simulink model "Feeder_1"  (Simulink 8.8)
settings: Solver=ode4  StartTime=0.0  StopTime=inf  FixedStep=Ts  RelTol=1e-3  EnableMultiTasking=on
PreLoadFcn:
  | Ts=125e-6;Core_Num = 0; np=1; nq=1; Vmin=.9;
PostLoadFcn:
  | Ts=125e-6;Core_Num = 0; np=1; nq=1; Vmin=.9;
InitFcn:
  | Ts=125e-6;Core_Num = 0; np=1; nq=1; Vmin=.9;
undefined symbols (not defined in the file or in its folder): another_event_name, DiscIntNeverNeededParam, I, j, Left, my_event_name, Right, type, V, X
libraries: powerlib x316, powerlib_meascontrol x227, simulink_extras x78, simulink x25, rtio_generic_c37_118 x22, ssn_lib x9, rtlab x6, powerlib_extras x3, artemis x1, rtio_opalrt_ml605ex1 x1, rtio_spectracom x1, rtio_generic_ethernet x1
(part 3 of 14)

== system Feeder_1/SS_DBUS ==
  DATATX : Inport
  Display : Display
  Ethernet  communication  interface : rtio_generic_ethernet/Ethernet communication interface  ctrl_id=1  nbr_to_remote_endpoint=64  type_to_remote_endpoint=FLOAT  offset_to_remote_endpoint=0  swap_tx=on  nbr_from_remote_endpoint=62  type_from_remote_endpoint=FLOAT  offset_from_remote_endpoint=0  swap_rx=on  exe_name='AsyncEthernet'  nic_name='eth0'  protocol=TCP  tcp_mode=Client  port=6340  remote_ip='10.1.2.2'
  OpComm : rtlab/OpComm  nbport=1  groupe_acq=1  subsys_rate=0  st=0  Synchronization=on  Interpolation=on  Threshold=1.0  Missed_Data=off  Sim_Time=off  Samples=off  dynSigOut=off  from_console=0  warning_done=off  writeOpCommFile=off  Offset=off
  Pulse input : DiscretePulseGenerator  Period=round(1/Ts)  SampleTime=Ts
  Terminator2 : Terminator
  DATARX : Outport
  PQIN : Outport  Port=2
  wires:
  Ethernet  communication  interface/2 -> Terminator2/1
  Pulse input/1 -> Ethernet  communication  interface/1
  DATATX/1 -> OpComm/1
  Ethernet  communication  interface/1 -> PQIN/1, DATARX/1
  OpComm/1 -> Display/1, Ethernet  communication  interface/2

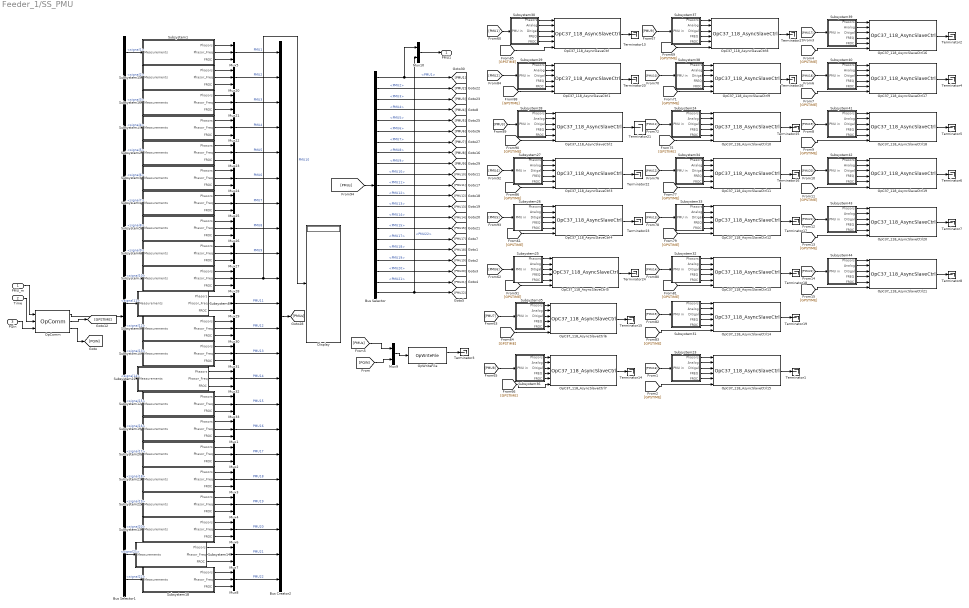
== system Feeder_1/SS_PMU ==
  PMU_m : Inport
  Time : Inport  Port=2
  PQin : Inport  Port=3
  Bus Creator2 : BusCreator  Inputs=22
  Bus Selector : BusSelector  OutputSignals=PMU1,PMU2,PMU3,PMU4,PMU5,PMU6,PMU7,PMU8,PMU9,PMU10,PMU11,PMU12,PMU13,PMU14,PMU15,PMU17,PMU18,PMU19,PMU20,PMU21,PMU22
  Bus Selector1 : BusSelector  OutputSignals=signal1,signal2,signal3,signal4,signal5,signal6,signal7,signal8,signal9,signal10,signal11,signal12,signal13,signal14,signal15,signal16,signal17,signal18,signal19,signal20,signal21,signal22
  Display : Display
  Mux{1..8,20..33} (22 alike) : Mux  Inputs=3
  Mux10 : Mux  Inputs=2
  Mux9 : Mux  Inputs=2
  OpC37_118_AsyncSlaveCtrl : rtio_generic_c37_118/OpC37_118_AsyncSlaveCtrl  dev_id=1  pmu_name='PMU1'  core_nbr=0  exe_name='AsyncC37_118_Slave'  nic_name='eth2'  proto=TCP  udp_port=7501  ip_addr_local='10.1.6.88'  port_local=7518  nominal_freq=60 Hz  data_rate_50=50  data_rate_60=30  timebase=1000000  ts_in=on  cfg_name='pmu_in_cfg.xml'
  OpC37_118_AsyncSlaveCtrl1 : rtio_generic_c37_118/OpC37_118_AsyncSlaveCtrl  dev_id=2  pmu_name='PMU2'  core_nbr=0  exe_name='AsyncC37_118_Slave'  nic_name='eth2'  proto=TCP  udp_port=7502  ip_addr_local='10.1.6.89'  port_local=7519  nominal_freq=60 Hz  data_rate_50=50  data_rate_60=30  timebase=1000000  ts_in=on  cfg_name='pmu_in_cfg.xml'
  OpC37_118_AsyncSlaveCtrl10 : rtio_generic_c37_118/OpC37_118_AsyncSlaveCtrl  dev_id=11  pmu_name='PMU11'  core_nbr=0  exe_name='AsyncC37_118_Slave'  nic_name='eth2'  proto=TCP  udp_port=7511  ip_addr_local='10.1.6.98'  port_local=7528  nominal_freq=60 Hz  data_rate_50=50  data_rate_60=30  timebase=1000000  ts_in=on  cfg_name='pmu_in_cfg.xml'
  OpC37_118_AsyncSlaveCtrl11 : rtio_generic_c37_118/OpC37_118_AsyncSlaveCtrl  dev_id=12  pmu_name='PMU12'  core_nbr=0  exe_name='AsyncC37_118_Slave'  nic_name='eth2'  proto=TCP  udp_port=7512  ip_addr_local='10.1.6.99'  port_local=7529  nominal_freq=60 Hz  data_rate_50=50  data_rate_60=30  timebase=1000000  ts_in=on  cfg_name='pmu_in_cfg.xml'
  OpC37_118_AsyncSlaveCtrl12 : rtio_generic_c37_118/OpC37_118_AsyncSlaveCtrl  dev_id=13  pmu_name='PMU13'  core_nbr=0  exe_name='AsyncC37_118_Slave'  nic_name='eth2'  proto=TCP  udp_port=7513  ip_addr_local='10.1.6.100'  port_local=7530  nominal_freq=60 Hz  data_rate_50=50  data_rate_60=30  timebase=1000000  ts_in=on  cfg_name='pmu_in_cfg.xml'
  OpC37_118_AsyncSlaveCtrl13 : rtio_generic_c37_118/OpC37_118_AsyncSlaveCtrl  dev_id=14  pmu_name='PMU14'  core_nbr=0  exe_name='AsyncC37_118_Slave'  nic_name='eth2'  proto=TCP  udp_port=7514  ip_addr_local='10.1.6.101'  port_local=7531  nominal_freq=60 Hz  data_rate_50=50  data_rate_60=30  timebase=1000000  ts_in=on  cfg_name='pmu_in_cfg.xml'
  OpC37_118_AsyncSlaveCtrl14 : rtio_generic_c37_118/OpC37_118_AsyncSlaveCtrl  dev_id=15  pmu_name='PMU15'  core_nbr=0  exe_name='AsyncC37_118_Slave'  nic_name='eth2'  proto=TCP  udp_port=7515  ip_addr_local='10.1.6.102'  port_local=7532  nominal_freq=60 Hz  data_rate_50=50  data_rate_60=30  timebase=1000000  ts_in=on  cfg_name='pmu_in_cfg.xml'
  OpC37_118_AsyncSlaveCtrl15 : rtio_generic_c37_118/OpC37_118_AsyncSlaveCtrl  dev_id=16  pmu_name='PMU16'  core_nbr=0  exe_name='AsyncC37_118_Slave'  nic_name='eth2'  proto=TCP  udp_port=7515  ip_addr_local='10.1.6.103'  port_local=7533  nominal_freq=60 Hz  data_rate_50=50  data_rate_60=30  timebase=1000000  ts_in=on  cfg_name='pmu_in_cfg.xml'
  OpC37_118_AsyncSlaveCtrl16 : rtio_generic_c37_118/OpC37_118_AsyncSlaveCtrl  dev_id=17  pmu_name='PMU17'  core_nbr=0  exe_name='AsyncC37_118_Slave'  nic_name='eth2'  proto=TCP  udp_port=7515  ip_addr_local='10.1.6.104'  port_local=7534  nominal_freq=60 Hz  data_rate_50=50  data_rate_60=30  timebase=1000000  ts_in=on  cfg_name='pmu_in_cfg.xml'
  OpC37_118_AsyncSlaveCtrl17 : rtio_generic_c37_118/OpC37_118_AsyncSlaveCtrl  dev_id=18  pmu_name='PMU18'  core_nbr=0  exe_name='AsyncC37_118_Slave'  nic_name='eth2'  proto=TCP  udp_port=7515  ip_addr_local='10.1.6.105'  port_local=7535  nominal_freq=60 Hz  data_rate_50=50  data_rate_60=30  timebase=1000000  ts_in=on  cfg_name='pmu_in_cfg.xml'
  OpC37_118_AsyncSlaveCtrl18 : rtio_generic_c37_118/OpC37_118_AsyncSlaveCtrl  dev_id=19  pmu_name='PMU19'  core_nbr=0  exe_name='AsyncC37_118_Slave'  nic_name='eth2'  proto=TCP  udp_port=7515  ip_addr_local='10.1.6.106'  port_local=7536  nominal_freq=60 Hz  data_rate_50=50  data_rate_60=30  timebase=1000000  ts_in=on  cfg_name='pmu_in_cfg.xml'
  OpC37_118_AsyncSlaveCtrl19 : rtio_generic_c37_118/OpC37_118_AsyncSlaveCtrl  dev_id=20  pmu_name='PMU20'  core_nbr=0  exe_name='AsyncC37_118_Slave'  nic_name='eth2'  proto=TCP  udp_port=7515  ip_addr_local='10.1.6.107'  port_local=7537  nominal_freq=60 Hz  data_rate_50=50  data_rate_60=30  timebase=1000000  ts_in=on  cfg_name='pmu_in_cfg.xml'
  OpC37_118_AsyncSlaveCtrl2 : rtio_generic_c37_118/OpC37_118_AsyncSlaveCtrl  dev_id=3  pmu_name='PMU3'  core_nbr=0  exe_name='AsyncC37_118_Slave'  nic_name='eth2'  proto=TCP  udp_port=7503  ip_addr_local='10.1.6.90'  port_local=7520  nominal_freq=60 Hz  data_rate_50=50  data_rate_60=30  timebase=1000000  ts_in=on  cfg_name='pmu_in_cfg.xml'
  OpC37_118_AsyncSlaveCtrl20 : rtio_generic_c37_118/OpC37_118_AsyncSlaveCtrl  dev_id=21  pmu_name='PMU21'  core_nbr=0  exe_name='AsyncC37_118_Slave'  nic_name='eth2'  proto=TCP  udp_port=7515  ip_addr_local='10.1.6.108'  port_local=7538  nominal_freq=60 Hz  data_rate_50=50  data_rate_60=30  timebase=1000000  ts_in=on  cfg_name='pmu_in_cfg.xml'
  OpC37_118_AsyncSlaveCtrl21 : rtio_generic_c37_118/OpC37_118_AsyncSlaveCtrl  dev_id=22  pmu_name='PMU22'  core_nbr=0  exe_name='AsyncC37_118_Slave'  nic_name='eth2'  proto=TCP  udp_port=7515  ip_addr_local='10.1.6.109'  port_local=7539  nominal_freq=60 Hz  data_rate_50=50  data_rate_60=30  timebase=1000000  ts_in=on  cfg_name='pmu_in_cfg.xml'
  OpC37_118_AsyncSlaveCtrl3 : rtio_generic_c37_118/OpC37_118_AsyncSlaveCtrl  dev_id=4  pmu_name='PMU4'  core_nbr=0  exe_name='AsyncC37_118_Slave'  nic_name='eth2'  proto=TCP  udp_port=7504  ip_addr_local='10.1.6.91'  port_local=7521  nominal_freq=60 Hz  data_rate_50=50  data_rate_60=30  timebase=1000000  ts_in=on  cfg_name='pmu_in_cfg.xml'
  OpC37_118_AsyncSlaveCtrl4 : rtio_generic_c37_118/OpC37_118_AsyncSlaveCtrl  dev_id=5  pmu_name='PMU5'  core_nbr=0  exe_name='AsyncC37_118_Slave'  nic_name='eth2'  proto=TCP  udp_port=7505  ip_addr_local='10.1.6.92'  port_local=7522  nominal_freq=60 Hz  data_rate_50=50  data_rate_60=30  timebase=1000000  ts_in=on  cfg_name='pmu_in_cfg.xml'
  OpC37_118_AsyncSlaveCtrl5 : rtio_generic_c37_118/OpC37_118_AsyncSlaveCtrl  dev_id=6  pmu_name='PMU6'  core_nbr=0  exe_name='AsyncC37_118_Slave'  nic_name='eth2'  proto=TCP  udp_port=7506  ip_addr_local='10.1.6.93'  port_local=7523  nominal_freq=60 Hz  data_rate_50=50  data_rate_60=30  timebase=1000000  ts_in=on  cfg_name='pmu_in_cfg.xml'
  OpC37_118_AsyncSlaveCtrl6 : rtio_generic_c37_118/OpC37_118_AsyncSlaveCtrl  dev_id=7  pmu_name='PMU7'  core_nbr=0  exe_name='AsyncC37_118_Slave'  nic_name='eth2'  proto=TCP  udp_port=7507  ip_addr_local='10.1.6.94'  port_local=7524  nominal_freq=60 Hz  data_rate_50=50  data_rate_60=30  timebase=1000000  ts_in=on  cfg_name='pmu_in_cfg.xml'
  OpC37_118_AsyncSlaveCtrl7 : rtio_generic_c37_118/OpC37_118_AsyncSlaveCtrl  dev_id=8  pmu_name='PMU8'  core_nbr=0  exe_name='AsyncC37_118_Slave'  nic_name='eth2'  proto=TCP  udp_port=7508  ip_addr_local='10.1.6.95'  port_local=7525  nominal_freq=60 Hz  data_rate_50=50  data_rate_60=30  timebase=1000000  ts_in=on  cfg_name='pmu_in_cfg.xml'
  OpC37_118_AsyncSlaveCtrl8 : rtio_generic_c37_118/OpC37_118_AsyncSlaveCtrl  dev_id=9  pmu_name='PMU9'  core_nbr=0  exe_name='AsyncC37_118_Slave'  nic_name='eth2'  proto=TCP  udp_port=7509  ip_addr_local='10.1.6.96'  port_local=7526  nominal_freq=60 Hz  data_rate_50=50  data_rate_60=30  timebase=1000000  ts_in=on  cfg_name='pmu_in_cfg.xml'
  OpC37_118_AsyncSlaveCtrl9 : rtio_generic_c37_118/OpC37_118_AsyncSlaveCtrl  dev_id=10  pmu_name='PMU10'  core_nbr=0  exe_name='AsyncC37_118_Slave'  nic_name='eth2'  proto=TCP  udp_port=7510  ip_addr_local='10.1.6.97'  port_local=7527  nominal_freq=60 Hz  data_rate_50=50  data_rate_60=30  timebase=1000000  ts_in=on  cfg_name='pmu_in_cfg.xml'
  OpComm : rtlab/OpComm  nbport=3  groupe_acq=1  subsys_rate=0  st=0  Synchronization=on  Interpolation=on  Threshold=1.0  Missed_Data=off  Sim_Time=off  Samples=off  dynSigOut=off  from_console=0  warning_done=off  writeOpCommFile=off  Offset=off
  OpWriteFile : rtlab/DataLogging/OpWriteFile  Static_File=on  varname=Baseline  Filename=Energise.mat  rtpath='./'  nrtpath='E:\Models\LOHO13_GT_DBUS\Results\Testdata'  Acq_Group=30  file_size=38092800  write_offline=off  Sim_Mode=off  Nb_Samples=800  Buffer_size=2374400
      settings: Decimation=10000
  Subsystem1 : Subsystem
  Subsystem10 : Subsystem
  Subsystem11 : Subsystem
  Subsystem12 : Subsystem
  Subsystem13 : Subsystem
  Subsystem14 : Subsystem
  Subsystem15 : Subsystem
  Subsystem16 : Subsystem
  Subsystem17 : Subsystem
  Subsystem18 : Subsystem
  Subsystem19 : Subsystem
  Subsystem2 : Subsystem
  Subsystem20 : Subsystem
  Subsystem21 : Subsystem
  Subsystem22 : Subsystem
  Subsystem23 : Subsystem
  Subsystem24 : Subsystem
  Subsystem25 : Subsystem
  Subsystem26 : Subsystem
  Subsystem27 : Subsystem
  Subsystem28 : Subsystem
  Subsystem29 : Subsystem
  Subsystem3 : Subsystem
  Subsystem30 : Subsystem
  Subsystem31 : Subsystem
  Subsystem32 : Subsystem
  Subsystem33 : Subsystem
  Subsystem34 : Subsystem
  Subsystem35 : Subsystem
  Subsystem36 : Subsystem
  Subsystem37 : Subsystem
  Subsystem38 : Subsystem
  Subsystem39 : Subsystem
  Subsystem4 : Subsystem
  Subsystem40 : Subsystem
  Subsystem41 : Subsystem
  Subsystem42 : Subsystem
  Subsystem43 : Subsystem
  Subsystem44 : Subsystem
  Subsystem5 : Subsystem
  Subsystem6 : Subsystem
  Subsystem7 : Subsystem
  Subsystem8 : Subsystem
  Subsystem9 : Subsystem
  Terminator{1..8,13..27} (23 alike) : Terminator
  PMU1 : Outport
  wires:
  [GPSTIME] -> OpC37_118_AsyncSlaveCtrl/6
  [GPSTIME] -> OpC37_118_AsyncSlaveCtrl1/6
  [GPSTIME] -> OpC37_118_AsyncSlaveCtrl2/6
  [GPSTIME] -> OpC37_118_AsyncSlaveCtrl3/6
  [GPSTIME] -> OpC37_118_AsyncSlaveCtrl4/6
  [GPSTIME] -> OpC37_118_AsyncSlaveCtrl5/6
  [GPSTIME] -> OpC37_118_AsyncSlaveCtrl6/6
  [GPSTIME] -> OpC37_118_AsyncSlaveCtrl7/6
  [GPSTIME] -> OpC37_118_AsyncSlaveCtrl8/6
  [GPSTIME] -> OpC37_118_AsyncSlaveCtrl9/6
  [GPSTIME] -> OpC37_118_AsyncSlaveCtrl10/6
  [GPSTIME] -> OpC37_118_AsyncSlaveCtrl11/6
  [GPSTIME] -> OpC37_118_AsyncSlaveCtrl12/6
  [GPSTIME] -> OpC37_118_AsyncSlaveCtrl13/6
  [GPSTIME] -> OpC37_118_AsyncSlaveCtrl14/6
  Subsystem31/1(Phasors) -> OpC37_118_AsyncSlaveCtrl14/1
  Subsystem31/2(Analog) -> OpC37_118_AsyncSlaveCtrl14/2
  Subsystem31/3(Ditigal) -> OpC37_118_AsyncSlaveCtrl14/3
  Subsystem31/4(FREQ) -> OpC37_118_AsyncSlaveCtrl14/4
  Subsystem31/5(FROC) -> OpC37_118_AsyncSlaveCtrl14/5
  [PMU15] -> Subsystem31/1(PMU in)
  Subsystem32/1(Phasors) -> OpC37_118_AsyncSlaveCtrl13/1
  Subsystem32/2(Analog) -> OpC37_118_AsyncSlaveCtrl13/2
  Subsystem32/3(Ditigal) -> OpC37_118_AsyncSlaveCtrl13/3
  Subsystem32/4(FREQ) -> OpC37_118_AsyncSlaveCtrl13/4
  Subsystem32/5(FROC) -> OpC37_118_AsyncSlaveCtrl13/5
  [PMU14] -> Subsystem32/1(PMU in)
  Subsystem33/1(Phasors) -> OpC37_118_AsyncSlaveCtrl12/1
  Subsystem33/2(Analog) -> OpC37_118_AsyncSlaveCtrl12/2
  Subsystem33/3(Ditigal) -> OpC37_118_AsyncSlaveCtrl12/3
  Subsystem33/4(FREQ) -> OpC37_118_AsyncSlaveCtrl12/4
  Subsystem33/5(FROC) -> OpC37_118_AsyncSlaveCtrl12/5
  [PMU13] -> Subsystem33/1(PMU in)
  Subsystem34/1(Phasors) -> OpC37_118_AsyncSlaveCtrl11/1
  Subsystem34/2(Analog) -> OpC37_118_AsyncSlaveCtrl11/2
  Subsystem34/3(Ditigal) -> OpC37_118_AsyncSlaveCtrl11/3
  Subsystem34/4(FREQ) -> OpC37_118_AsyncSlaveCtrl11/4
  Subsystem34/5(FROC) -> OpC37_118_AsyncSlaveCtrl11/5
  [PMU12] -> Subsystem34/1(PMU in)
  Subsystem35/1(Phasors) -> OpC37_118_AsyncSlaveCtrl6/1
  Subsystem35/2(Analog) -> OpC37_118_AsyncSlaveCtrl6/2
  Subsystem35/3(Ditigal) -> OpC37_118_AsyncSlaveCtrl6/3
  Subsystem35/4(FREQ) -> OpC37_118_AsyncSlaveCtrl6/4
  Subsystem35/5(FROC) -> OpC37_118_AsyncSlaveCtrl6/5
  [PMU7] -> Subsystem35/1(PMU in)
  Subsystem36/1(Phasors) -> OpC37_118_AsyncSlaveCtrl7/1
  Subsystem36/2(Analog) -> OpC37_118_AsyncSlaveCtrl7/2
  Subsystem36/3(Ditigal) -> OpC37_118_AsyncSlaveCtrl7/3
  Subsystem36/4(FREQ) -> OpC37_118_AsyncSlaveCtrl7/4
  Subsystem36/5(FROC) -> OpC37_118_AsyncSlaveCtrl7/5
  [PMU8] -> Subsystem36/1(PMU in)
  Subsystem37/1(Phasors) -> OpC37_118_AsyncSlaveCtrl8/1
  Subsystem37/2(Analog) -> OpC37_118_AsyncSlaveCtrl8/2
  Subsystem37/3(Ditigal) -> OpC37_118_AsyncSlaveCtrl8/3
  Subsystem37/4(FREQ) -> OpC37_118_AsyncSlaveCtrl8/4
  Subsystem37/5(FROC) -> OpC37_118_AsyncSlaveCtrl8/5
  [PMU9] -> Subsystem37/1(PMU in)
  Subsystem38/1(Phasors) -> OpC37_118_AsyncSlaveCtrl9/1
  Subsystem38/2(Analog) -> OpC37_118_AsyncSlaveCtrl9/2
  Subsystem38/3(Ditigal) -> OpC37_118_AsyncSlaveCtrl9/3
  Subsystem38/4(FREQ) -> OpC37_118_AsyncSlaveCtrl9/4
  Subsystem38/5(FROC) -> OpC37_118_AsyncSlaveCtrl9/5
  [PMU10] -> Subsystem38/1(PMU in)
  Subsystem24/1(Phasors) -> OpC37_118_AsyncSlaveCtrl10/1
  Subsystem24/2(Analog) -> OpC37_118_AsyncSlaveCtrl10/2
  Subsystem24/3(Ditigal) -> OpC37_118_AsyncSlaveCtrl10/3
  Subsystem24/4(FREQ) -> OpC37_118_AsyncSlaveCtrl10/4
  Subsystem24/5(FROC) -> OpC37_118_AsyncSlaveCtrl10/5
  [PMU11] -> Subsystem24/1(PMU in)
  Subsystem25/1(Phasors) -> OpC37_118_AsyncSlaveCtrl5/1
  Subsystem25/2(Analog) -> OpC37_118_AsyncSlaveCtrl5/2
  Subsystem25/3(Ditigal) -> OpC37_118_AsyncSlaveCtrl5/3
  Subsystem25/4(FREQ) -> OpC37_118_AsyncSlaveCtrl5/4
  Subsystem25/5(FROC) -> OpC37_118_AsyncSlaveCtrl5/5
  [PMU6] -> Subsystem25/1(PMU in)
  Subsystem26/1(Phasors) -> OpC37_118_AsyncSlaveCtrl4/1
  Subsystem26/2(Analog) -> OpC37_118_AsyncSlaveCtrl4/2
  Subsystem26/3(Ditigal) -> OpC37_118_AsyncSlaveCtrl4/3
  Subsystem26/4(FREQ) -> OpC37_118_AsyncSlaveCtrl4/4
  Subsystem26/5(FROC) -> OpC37_118_AsyncSlaveCtrl4/5
  [PMU5] -> Subsystem26/1(PMU in)
  Subsystem27/1(Phasors) -> OpC37_118_AsyncSlaveCtrl3/1
  Subsystem27/2(Analog) -> OpC37_118_AsyncSlaveCtrl3/2
  Subsystem27/3(Ditigal) -> OpC37_118_AsyncSlaveCtrl3/3
  Subsystem27/4(FREQ) -> OpC37_118_AsyncSlaveCtrl3/4
  Subsystem27/5(FROC) -> OpC37_118_AsyncSlaveCtrl3/5
  [PMU4] -> Subsystem27/1(PMU in)
  Subsystem28/1(Phasors) -> OpC37_118_AsyncSlaveCtrl2/1
  Subsystem28/2(Analog) -> OpC37_118_AsyncSlaveCtrl2/2
  Subsystem28/3(Ditigal) -> OpC37_118_AsyncSlaveCtrl2/3
  Subsystem28/4(FREQ) -> OpC37_118_AsyncSlaveCtrl2/4
  Subsystem28/5(FROC) -> OpC37_118_AsyncSlaveCtrl2/5
  [PMU3] -> Subsystem28/1(PMU in)
  Subsystem29/1(Phasors) -> OpC37_118_AsyncSlaveCtrl1/1
  Subsystem29/2(Analog) -> OpC37_118_AsyncSlaveCtrl1/2
  Subsystem29/3(Ditigal) -> OpC37_118_AsyncSlaveCtrl1/3
  Subsystem29/4(FREQ) -> OpC37_118_AsyncSlaveCtrl1/4
  Subsystem29/5(FROC) -> OpC37_118_AsyncSlaveCtrl1/5
  [PMU2] -> Subsystem29/1(PMU in)
  Subsystem30/1(Phasors) -> OpC37_118_AsyncSlaveCtrl/1
  Subsystem30/2(Analog) -> OpC37_118_AsyncSlaveCtrl/2
  Subsystem30/3(Ditigal) -> OpC37_118_AsyncSlaveCtrl/3
  Subsystem30/4(FREQ) -> OpC37_118_AsyncSlaveCtrl/4
  Subsystem30/5(FROC) -> OpC37_118_AsyncSlaveCtrl/5
  [PMU1] -> Subsystem30/1(PMU in)
  Bus Selector/2 -> [PMU2]  "<PMU2>"
  Bus Selector/3 -> [PMU3]  "<PMU3>"
  Bus Selector/5 -> [PMU5]  "<PMU5>"
  Bus Selector/7 -> [PMU7]  "<PMU7>"
  Bus Selector/9 -> [PMU9]  "<PMU9>"
  Bus Selector/11 -> [PMU11]  "<PMU11>"
  Bus Selector/13 -> [PMU13]  "<PMU13>"
  Bus Selector/15 -> [PMU15]  "<PMU15>"
  OpC37_118_AsyncSlaveCtrl/1 -> Terminator13/1
  OpC37_118_AsyncSlaveCtrl1/1 -> Terminator20/1
  OpC37_118_AsyncSlaveCtrl2/1 -> Terminator21/1
  OpC37_118_AsyncSlaveCtrl3/1 -> Terminator22/1
  OpC37_118_AsyncSlaveCtrl4/1 -> Terminator23/1
  OpC37_118_AsyncSlaveCtrl5/1 -> Terminator24/1
  OpC37_118_AsyncSlaveCtrl10/1 -> Terminator25/1
  OpC37_118_AsyncSlaveCtrl9/1 -> Terminator26/1
  OpC37_118_AsyncSlaveCtrl8/1 -> Terminator27/1
  OpC37_118_AsyncSlaveCtrl7/1 -> Terminator14/1
  OpC37_118_AsyncSlaveCtrl6/1 -> Terminator15/1
  OpC37_118_AsyncSlaveCtrl11/1 -> Terminator16/1
  OpC37_118_AsyncSlaveCtrl12/1 -> Terminator17/1
  OpC37_118_AsyncSlaveCtrl13/1 -> Terminator18/1
  OpC37_118_AsyncSlaveCtrl14/1 -> Terminator19/1
  PMU_m/1 -> OpComm/1
  Time/1 -> OpComm/2
  OpComm/2 -> [GPSTIME]
  Subsystem1/1(Phasors) -> Mux5/1
  Subsystem1/2(Phasor_Freq) -> Mux5/2
  Subsystem1/3(FROC) -> Mux5/3
  Subsystem15/1(Phasors) -> Mux20/1
  Subsystem15/2(Phasor_Freq) -> Mux20/2
  Subsystem15/3(FROC) -> Mux20/3
  Subsystem16/1(Phasors) -> Mux21/1
  Mux33/1 -> Bus Creator2/15  "PMU15"
  Mux32/1 -> Bus Creator2/14  "PMU14"
  Mux31/1 -> Bus Creator2/13  "PMU13"
  Mux30/1 -> Bus Creator2/12  "PMU12"
  Mux29/1 -> Bus Creator2/11  "PMU11"
  Mux5/1 -> Bus Creator2/1  "PMU1"
  Mux20/1 -> Bus Creator2/2  "PMU2"
  Mux21/1 -> Bus Creator2/3  "PMU3"
  Mux22/1 -> Bus Creator2/4  "PMU4"
  Mux23/1 -> Bus Creator2/5  "PMU5"
  Mux24/1 -> Bus Creator2/6  "PMU6"
  Mux25/1 -> Bus Creator2/7  "PMU7"
  Mux27/1 -> Bus Creator2/9  "PMU9"
  Mux28/1 -> Display/1, Bus Creator2/10  "PMU10"
  Mux26/1 -> Bus Creator2/8  "PMU8"
  Subsystem16/2(Phasor_Freq) -> Mux21/2
  Subsystem16/3(FROC) -> Mux21/3
  Subsystem17/1(Phasors) -> Mux22/1
  Subsystem17/2(Phasor_Freq) -> Mux22/2
  Subsystem17/3(FROC) -> Mux22/3
  Subsystem2/1(Phasors) -> Mux23/1
  Subsystem2/3(FROC) -> Mux23/3
  Subsystem2/2(Phasor_Freq) -> Mux23/2
  Subsystem3/1(Phasors) -> Mux24/1
  Subsystem3/2(Phasor_Freq) -> Mux24/2
  Subsystem3/3(FROC) -> Mux24/3
  Subsystem4/1(Phasors) -> Mux25/1
  Subsystem4/2(Phasor_Freq) -> Mux25/2
  Subsystem4/3(FROC) -> Mux25/3
  Subsystem5/1(Phasors) -> Mux26/1
  Subsystem5/2(Phasor_Freq) -> Mux26/2
  Subsystem5/3(FROC) -> Mux26/3
  Subsystem6/1(Phasors) -> Mux27/1
  Subsystem6/2(Phasor_Freq) -> Mux27/2
  Subsystem6/3(FROC) -> Mux27/3
  Subsystem7/1(Phasors) -> Mux28/1
  Subsystem7/2(Phasor_Freq) -> Mux28/2
  Subsystem7/3(FROC) -> Mux28/3
  Subsystem8/1(Phasors) -> Mux29/1
  Subsystem8/2(Phasor_Freq) -> Mux29/2
  Subsystem8/3(FROC) -> Mux29/3
  Subsystem9/1(Phasors) -> Mux30/1
  Subsystem9/2(Phasor_Freq) -> Mux30/2
  Subsystem9/3(FROC) -> Mux30/3
  Subsystem10/1(Phasors) -> Mux31/1
  Subsystem10/2(Phasor_Freq) -> Mux31/2
  Subsystem10/3(FROC) -> Mux31/3
  Subsystem11/1(Phasors) -> Mux32/1
  Subsystem11/2(Phasor_Freq) -> Mux32/2
  Subsystem11/3(FROC) -> Mux32/3
  Subsystem12/1(Phasors) -> Mux33/1
  Subsystem12/2(Phasor_Freq) -> Mux33/2
  Subsystem12/3(FROC) -> Mux33/3
  Bus Selector1/1 -> Subsystem1/1(Measurements)  "<signal1>"
  Bus Selector1/2 -> Subsystem15/1(Measurements)  "<signal2>"
  Bus Selector1/3 -> Subsystem16/1(Measurements)  "<signal3>"
  Bus Selector1/4 -> Subsystem17/1(Measurements)  "<signal4>"
  Bus Selector1/5 -> Subsystem2/1(Measurements)  "<signal5>"
  Bus Selector1/6 -> Subsystem3/1(Measurements)  "<signal6>"
  Bus Selector1/7 -> Subsystem4/1(Measurements)  "<signal7>"
  Bus Selector1/8 -> Subsystem5/1(Measurements)  "<signal8>"
  Bus Selector1/9 -> Subsystem6/1(Measurements)  "<signal9>"
  Bus Selector1/10 -> Subsystem7/1(Measurements)  "<signal10>"
  Bus Selector1/11 -> Subsystem8/1(Measurements)  "<signal11>"
  Bus Selector1/12 -> Subsystem9/1(Measurements)  "<signal12>"
  Bus Selector1/13 -> Subsystem10/1(Measurements)  "<signal13>"
  Bus Selector1/14 -> Subsystem11/1(Measurements)  "<signal14>"
  Bus Selector1/15 -> Subsystem12/1(Measurements)  "<signal15>"
  OpComm/1 -> Bus Selector1/1
  Bus Creator2/1 -> [PMUs]
  [PMUs] -> Bus Selector/1
  Bus Selector/4 -> [PMU4]  "<PMU4>"
  Bus Selector/6 -> [PMU6]  "<PMU6>"
  Bus Selector/8 -> [PMU8]  "<PMU8>"
  Bus Selector/10 -> [PMU10]  "<PMU10>"
  Bus Selector/12 -> [PMU12]  "<PMU12>"
  Bus Selector/14 -> [PMU14]  "<PMU14>"
  Bus Selector/1 -> Mux10/1, [PMU1]  "<PMU1>"
  OpWriteFile/1 -> Terminator3/1
  Bus Selector1/22 -> Subsystem18/1(Measurements)  "<signal22>"
  Bus Selector1/21 -> Subsystem14/1(Measurements)  "<signal21>"
  Bus Selector1/20 -> Subsystem13/1(Measurements)  "<signal20>"
  Bus Selector1/19 -> Subsystem22/1(Measurements)  "<signal19>"
  Bus Selector1/18 -> Subsystem21/1(Measurements)  "<signal18>"
  Bus Selector1/17 -> Subsystem20/1(Measurements)  "<signal17>"
  Bus Selector1/16 -> Subsystem19/1(Measurements)  "<signal16>"
  Mux8/1 -> Bus Creator2/22  "PMU22"
  Mux7/1 -> Bus Creator2/21  "PMU21"
  Mux6/1 -> Bus Creator2/20  "PMU20"
  Mux4/1 -> Bus Creator2/19  "PMU19"
  Mux3/1 -> Bus Creator2/18  "PMU18"
  Mux1/1 -> Bus Creator2/16  "PMU16"
  Mux2/1 -> Bus Creator2/17  "PMU17"
  Subsystem19/1(Phasors) -> Mux1/1
  Subsystem19/2(Phasor_Freq) -> Mux1/2
  Subsystem19/3(FROC) -> Mux1/3
  Subsystem20/1(Phasors) -> Mux2/1
  Subsystem20/2(Phasor_Freq) -> Mux2/2
  Subsystem20/3(FROC) -> Mux2/3
  Subsystem21/1(Phasors) -> Mux3/1
  Subsystem21/2(Phasor_Freq) -> Mux3/2
  Subsystem21/3(FROC) -> Mux3/3
  Subsystem22/1(Phasors) -> Mux4/1
  Subsystem22/2(Phasor_Freq) -> Mux4/2
  Subsystem22/3(FROC) -> Mux4/3
  Subsystem13/1(Phasors) -> Mux6/1
  Subsystem13/2(Phasor_Freq) -> Mux6/2
  Subsystem13/3(FROC) -> Mux6/3
  Subsystem14/1(Phasors) -> Mux7/1
  Subsystem14/2(Phasor_Freq) -> Mux7/2
  Subsystem14/3(FROC) -> Mux7/3
  Subsystem18/1(Phasors) -> Mux8/1
  Subsystem18/2(Phasor_Freq) -> Mux8/2
  Subsystem18/3(FROC) -> Mux8/3
  [GPSTIME] -> OpC37_118_AsyncSlaveCtrl15/6
  Subsystem23/1(Phasors) -> OpC37_118_AsyncSlaveCtrl15/1
  Subsystem23/2(Analog) -> OpC37_118_AsyncSlaveCtrl15/2
  Subsystem23/3(Ditigal) -> OpC37_118_AsyncSlaveCtrl15/3
  Subsystem23/4(FREQ) -> OpC37_118_AsyncSlaveCtrl15/4
  Subsystem23/5(FROC) -> OpC37_118_AsyncSlaveCtrl15/5
  [PMU16] -> Subsystem23/1(PMU in)
  OpC37_118_AsyncSlaveCtrl15/1 -> Terminator1/1
  [GPSTIME] -> OpC37_118_AsyncSlaveCtrl16/6
  Subsystem39/1(Phasors) -> OpC37_118_AsyncSlaveCtrl16/1
  Subsystem39/2(Analog) -> OpC37_118_AsyncSlaveCtrl16/2
  Subsystem39/3(Ditigal) -> OpC37_118_AsyncSlaveCtrl16/3
  Subsystem39/4(FREQ) -> OpC37_118_AsyncSlaveCtrl16/4
  Subsystem39/5(FROC) -> OpC37_118_AsyncSlaveCtrl16/5
  [PMU17] -> Subsystem39/1(PMU in)
  OpC37_118_AsyncSlaveCtrl16/1 -> Terminator2/1
  [GPSTIME] -> OpC37_118_AsyncSlaveCtrl17/6
  Subsystem40/1(Phasors) -> OpC37_118_AsyncSlaveCtrl17/1
  Subsystem40/2(Analog) -> OpC37_118_AsyncSlaveCtrl17/2
  Subsystem40/3(Ditigal) -> OpC37_118_AsyncSlaveCtrl17/3
  Subsystem40/4(FREQ) -> OpC37_118_AsyncSlaveCtrl17/4
  Subsystem40/5(FROC) -> OpC37_118_AsyncSlaveCtrl17/5
  [PMU18] -> Subsystem40/1(PMU in)
  OpC37_118_AsyncSlaveCtrl17/1 -> Terminator4/1
  [GPSTIME] -> OpC37_118_AsyncSlaveCtrl18/6
  Subsystem41/2(Analog) -> OpC37_118_AsyncSlaveCtrl18/2
  Subsystem41/3(Ditigal) -> OpC37_118_AsyncSlaveCtrl18/3
  Subsystem41/4(FREQ) -> OpC37_118_AsyncSlaveCtrl18/4
  Subsystem41/5(FROC) -> OpC37_118_AsyncSlaveCtrl18/5
  [PMU19] -> Subsystem41/1(PMU in)
  OpC37_118_AsyncSlaveCtrl18/1 -> Terminator5/1
  [GPSTIME] -> OpC37_118_AsyncSlaveCtrl19/6
  Subsystem42/2(Analog) -> OpC37_118_AsyncSlaveCtrl19/2
  Subsystem42/3(Ditigal) -> OpC37_118_AsyncSlaveCtrl19/3
  Subsystem42/4(FREQ) -> OpC37_118_AsyncSlaveCtrl19/4
  Subsystem42/5(FROC) -> OpC37_118_AsyncSlaveCtrl19/5
  [PMU20] -> Subsystem42/1(PMU in)
  OpC37_118_AsyncSlaveCtrl19/1 -> Terminator6/1
  Subsystem42/1(Phasors) -> OpC37_118_AsyncSlaveCtrl19/1
  Subsystem41/1(Phasors) -> OpC37_118_AsyncSlaveCtrl18/1
  [GPSTIME] -> OpC37_118_AsyncSlaveCtrl20/6
  Subsystem43/2(Analog) -> OpC37_118_AsyncSlaveCtrl20/2
  Subsystem43/3(Ditigal) -> OpC37_118_AsyncSlaveCtrl20/3
  Subsystem43/4(FREQ) -> OpC37_118_AsyncSlaveCtrl20/4
  Subsystem43/5(FROC) -> OpC37_118_AsyncSlaveCtrl20/5
  [PMU21] -> Subsystem43/1(PMU in)
  OpC37_118_AsyncSlaveCtrl20/1 -> Terminator7/1
  Subsystem43/1(Phasors) -> OpC37_118_AsyncSlaveCtrl20/1
  [GPSTIME] -> OpC37_118_AsyncSlaveCtrl21/6
  Subsystem44/2(Analog) -> OpC37_118_AsyncSlaveCtrl21/2
  Subsystem44/3(Ditigal) -> OpC37_118_AsyncSlaveCtrl21/3
  Subsystem44/4(FREQ) -> OpC37_118_AsyncSlaveCtrl21/4
  Subsystem44/5(FROC) -> OpC37_118_AsyncSlaveCtrl21/5
  [PMU22] -> Subsystem44/1(PMU in)
  OpC37_118_AsyncSlaveCtrl21/1 -> Terminator8/1
  Subsystem44/1(Phasors) -> OpC37_118_AsyncSlaveCtrl21/1
  Bus Selector/21 -> Mux10/2, [PMU22]  "<PMU22>"
  Bus Selector/20 -> [PMU21]  "<PMU21>"
  Bus Selector/19 -> [PMU20]  "<PMU20>"
  Bus Selector/18 -> [PMU19]  "<PMU19>"
  Bus Selector/17 -> [PMU18]  "<PMU18>"
  Bus Selector/16 -> [PMU17]  "<PMU17>"
  [PMUs] -> Mux9/1
  Mux9/1 -> OpWriteFile/1
  PQin/1 -> OpComm/3
  OpComm/3 -> [PQIN]
  [PQIN] -> Mux9/2
  Mux10/1 -> PMU1/1

== system Feeder_1/SM_NG/Dynamic Load BCDC2 ==
  P : Inport
  Q : Inport  Port=2
  Ground27 : powerlib/Elements/Ground  LConnTagsString=a
  Single-Phase Dynamic Load1 : Subsystem  DialogController=POWERSYS.PowerSysDialog  mask(Single-Phase Dynamic Load){NominalVoltage=|, ActiveReactivePowers=[934247.1199 467237.5312], PositiveSequence=[1 0], ExternalControl=on, NpNq=[np nq], TimeConstants=[0  0  0  0], MinimumVoltage=Vmin, LoadFlowParameters=[4,0,0,0,0]}
      mask NominalVoltage=|
      | [7967.4337
      | 60]
      mask prompts: NominalVoltage "Nominal voltage and frequency  [Vn(Vrms) fn(Hz)]:"; ActiveReactivePowers "Active and reactive power at initial voltage [Po(W) Qo(var)]:"; PositiveSequence "Initial voltage Vo [Mag(pu) Phase (deg.)]:"; ExternalControl "External control of PQ"; NpNq "Parameters [ np  nq ]:"; TimeConstants "Time constants [Tp1 Tp2 Tq1 Tq2]  (s):"; MinimumVoltage "Minimum voltage Vmin (pu):"; LoadFlowParameters "Load Flow parameters"
      mask help:
      | Implements a single-phase dynamic load. Active  power P and reactive
      | power Q absorbed by the load vary as function of voltage V  according to the
      | following equations:
      |
      |   If V>Vmin, P and Q vary as follows:
      |        P = Po * (V/Vo)^np * (1+Tp1.s)/(1+Tp2.s)
      |        Q = Qo * (V/Vo)^nq * (1+Tq1.s)/(1+Tq2.s)
      |   if V<Vmin
      |      Same equations with np=nq=2 (constant impedance load)
      mask init: same as Feeder_1/SM_NG/Single-Phase Dynamic Load32
      mask Help: helpview(psbhelp)
      mask Callback ExternalControl: powericon('ThreePhaseDynamicLoadCback',gcb);
      mask Display:
      | plot(-45,-45,45,45,[0,9,18,24,29,30,29,24,18,9,0,-9,-18,-24,-29,-30,-29,-24,-18,-9,0]*.9,[30,29,24,18,9,0,-9,-18,-24,-29,-30,-29,-24,-18,-9,0,9,18,24,29,30]*.9)
      | plot([0,0,10,0,-10,0]*1.1,[15,-5,-5,-15,-5,-5]*1.1)
  Single-Phase Dynamic Load2 : Subsystem  DialogController=POWERSYS.PowerSysDialog  mask(Single-Phase Dynamic Load){NominalVoltage=|, ActiveReactivePowers=[586764.5672 402164.5376], PositiveSequence=[1 0], ExternalControl=on, NpNq=[np nq], TimeConstants=[0  0  0  0], MinimumVoltage=Vmin, LoadFlowParameters=[4,0,0,0,0]}
      mask NominalVoltage=|
      | [7967.4337
      | 60]
      mask prompts: NominalVoltage "Nominal voltage and frequency  [Vn(Vrms) fn(Hz)]:"; ActiveReactivePowers "Active and reactive power at initial voltage [Po(W) Qo(var)]:"; PositiveSequence "Initial voltage Vo [Mag(pu) Phase (deg.)]:"; ExternalControl "External control of PQ"; NpNq "Parameters [ np  nq ]:"; TimeConstants "Time constants [Tp1 Tp2 Tq1 Tq2]  (s):"; MinimumVoltage "Minimum voltage Vmin (pu):"; LoadFlowParameters "Load Flow parameters"
      mask help:
      | Implements a single-phase dynamic load. Active  power P and reactive
      | power Q absorbed by the load vary as function of voltage V  according to the
      | following equations:
      |
      |   If V>Vmin, P and Q vary as follows:
      |        P = Po * (V/Vo)^np * (1+Tp1.s)/(1+Tp2.s)
      |        Q = Qo * (V/Vo)^nq * (1+Tq1.s)/(1+Tq2.s)
      |   if V<Vmin
      |      Same equations with np=nq=2 (constant impedance load)
      mask init: same as Feeder_1/SM_NG/Single-Phase Dynamic Load32
      mask Help: helpview(psbhelp)
      mask Callback ExternalControl: powericon('ThreePhaseDynamicLoadCback',gcb);
      mask Display:
      | plot(-45,-45,45,45,[0,9,18,24,29,30,29,24,18,9,0,-9,-18,-24,-29,-30,-29,-24,-18,-9,0]*.9,[30,29,24,18,9,0,-9,-18,-24,-29,-30,-29,-24,-18,-9,0,9,18,24,29,30]*.9)
      | plot([0,0,10,0,-10,0]*1.1,[15,-5,-5,-15,-5,-5]*1.1)
  Single-Phase Dynamic Load9 : Subsystem  DialogController=POWERSYS.PowerSysDialog  mask(Single-Phase Dynamic Load){NominalVoltage=|, ActiveReactivePowers=[473340.7231 336359.2548], PositiveSequence=[1 0], ExternalControl=on, NpNq=[np nq], TimeConstants=[0  0  0  0], MinimumVoltage=Vmin, LoadFlowParameters=[4,0,0,0,0]}
      mask NominalVoltage=|
      | [7967.4337
      | 60]
      mask prompts: NominalVoltage "Nominal voltage and frequency  [Vn(Vrms) fn(Hz)]:"; ActiveReactivePowers "Active and reactive power at initial voltage [Po(W) Qo(var)]:"; PositiveSequence "Initial voltage Vo [Mag(pu) Phase (deg.)]:"; ExternalControl "External control of PQ"; NpNq "Parameters [ np  nq ]:"; TimeConstants "Time constants [Tp1 Tp2 Tq1 Tq2]  (s):"; MinimumVoltage "Minimum voltage Vmin (pu):"; LoadFlowParameters "Load Flow parameters"
      mask help:
      | Implements a single-phase dynamic load. Active  power P and reactive
      | power Q absorbed by the load vary as function of voltage V  according to the
      | following equations:
      |
      |   If V>Vmin, P and Q vary as follows:
      |        P = Po * (V/Vo)^np * (1+Tp1.s)/(1+Tp2.s)
      |        Q = Qo * (V/Vo)^nq * (1+Tq1.s)/(1+Tq2.s)
      |   if V<Vmin
      |      Same equations with np=nq=2 (constant impedance load)
      mask init: same as Feeder_1/SM_NG/Single-Phase Dynamic Load32
      mask Help: helpview(psbhelp)
      mask Callback ExternalControl: powericon('ThreePhaseDynamicLoadCback',gcb);
      mask Display:
      | plot(-45,-45,45,45,[0,9,18,24,29,30,29,24,18,9,0,-9,-18,-24,-29,-30,-29,-24,-18,-9,0]*.9,[30,29,24,18,9,0,-9,-18,-24,-29,-30,-29,-24,-18,-9,0,9,18,24,29,30]*.9)
      | plot([0,0,10,0,-10,0]*1.1,[15,-5,-5,-15,-5,-5]*1.1)
  A : PMIOPort  Port=1  Side=Right
  B : PMIOPort  Port=2  Side=Right
  C : PMIOPort  Port=3  Side=Right
  wires:
  P/1 -> Single-Phase Dynamic Load2/1(P), Single-Phase Dynamic Load1/1(P), Single-Phase Dynamic Load9/1(P)
  Q/1 -> Single-Phase Dynamic Load1/2(Q), Single-Phase Dynamic Load2/2(Q), Single-Phase Dynamic Load9/2(Q)
  connections:
  Single-Phase Dynamic Load9/LConn2 -- Single-Phase Dynamic Load1/LConn2 -- Ground27/LConn1 -- Single-Phase Dynamic Load2/LConn2
  A/RConn1 -- Single-Phase Dynamic Load9/LConn1
  Single-Phase Dynamic Load2/LConn1 -- C/RConn1
  Single-Phase Dynamic Load1/LConn1 -- B/RConn1

== system Feeder_1/SM_NG/Dynamic Load BCDC3 ==
  P : Inport
  Q : Inport  Port=2
  Ground27 : powerlib/Elements/Ground  LConnTagsString=a
  Single-Phase Dynamic Load1 : Subsystem  DialogController=POWERSYS.PowerSysDialog  mask(Single-Phase Dynamic Load){NominalVoltage=|, ActiveReactivePowers=[359272.8363 164258.4315], PositiveSequence=[1 0], ExternalControl=on, NpNq=[np nq], TimeConstants=[0  0  0  0], MinimumVoltage=Vmin, LoadFlowParameters=[4,0,0,0,0]}
      mask NominalVoltage=|
      | [7967.4337
      | 60]
      mask prompts: NominalVoltage "Nominal voltage and frequency  [Vn(Vrms) fn(Hz)]:"; ActiveReactivePowers "Active and reactive power at initial voltage [Po(W) Qo(var)]:"; PositiveSequence "Initial voltage Vo [Mag(pu) Phase (deg.)]:"; ExternalControl "External control of PQ"; NpNq "Parameters [ np  nq ]:"; TimeConstants "Time constants [Tp1 Tp2 Tq1 Tq2]  (s):"; MinimumVoltage "Minimum voltage Vmin (pu):"; LoadFlowParameters "Load Flow parameters"
      mask help:
      | Implements a single-phase dynamic load. Active  power P and reactive
      | power Q absorbed by the load vary as function of voltage V  according to the
      | following equations:
      |
      |   If V>Vmin, P and Q vary as follows:
      |        P = Po * (V/Vo)^np * (1+Tp1.s)/(1+Tp2.s)
      |        Q = Qo * (V/Vo)^nq * (1+Tq1.s)/(1+Tq2.s)
      |   if V<Vmin
      |      Same equations with np=nq=2 (constant impedance load)
      mask init: same as Feeder_1/SM_NG/Single-Phase Dynamic Load32
      mask Help: helpview(psbhelp)
      mask Callback ExternalControl: powericon('ThreePhaseDynamicLoadCback',gcb);
      mask Display:
      | plot(-45,-45,45,45,[0,9,18,24,29,30,29,24,18,9,0,-9,-18,-24,-29,-30,-29,-24,-18,-9,0]*.9,[30,29,24,18,9,0,-9,-18,-24,-29,-30,-29,-24,-18,-9,0,9,18,24,29,30]*.9)
      | plot([0,0,10,0,-10,0]*1.1,[15,-5,-5,-15,-5,-5]*1.1)
  Single-Phase Dynamic Load2 : Subsystem  DialogController=POWERSYS.PowerSysDialog  mask(Single-Phase Dynamic Load){NominalVoltage=|, ActiveReactivePowers=[167826.2591 104736.8385], PositiveSequence=[1 0], ExternalControl=on, NpNq=[np nq], TimeConstants=[0  0  0  0], MinimumVoltage=Vmin, LoadFlowParameters=[4,0,0,0,0]}
      mask NominalVoltage=|
      | [7967.4337
      | 60]
      mask prompts: NominalVoltage "Nominal voltage and frequency  [Vn(Vrms) fn(Hz)]:"; ActiveReactivePowers "Active and reactive power at initial voltage [Po(W) Qo(var)]:"; PositiveSequence "Initial voltage Vo [Mag(pu) Phase (deg.)]:"; ExternalControl "External control of PQ"; NpNq "Parameters [ np  nq ]:"; TimeConstants "Time constants [Tp1 Tp2 Tq1 Tq2]  (s):"; MinimumVoltage "Minimum voltage Vmin (pu):"; LoadFlowParameters "Load Flow parameters"
      mask help:
      | Implements a single-phase dynamic load. Active  power P and reactive
      | power Q absorbed by the load vary as function of voltage V  according to the
      | following equations:
      |
      |   If V>Vmin, P and Q vary as follows:
      |        P = Po * (V/Vo)^np * (1+Tp1.s)/(1+Tp2.s)
      |        Q = Qo * (V/Vo)^nq * (1+Tq1.s)/(1+Tq2.s)
      |   if V<Vmin
      |      Same equations with np=nq=2 (constant impedance load)
      mask init: same as Feeder_1/SM_NG/Single-Phase Dynamic Load32
      mask Help: helpview(psbhelp)
      mask Callback ExternalControl: powericon('ThreePhaseDynamicLoadCback',gcb);
      mask Display:
      | plot(-45,-45,45,45,[0,9,18,24,29,30,29,24,18,9,0,-9,-18,-24,-29,-30,-29,-24,-18,-9,0]*.9,[30,29,24,18,9,0,-9,-18,-24,-29,-30,-29,-24,-18,-9,0,9,18,24,29,30]*.9)
      | plot([0,0,10,0,-10,0]*1.1,[15,-5,-5,-15,-5,-5]*1.1)
  Single-Phase Dynamic Load9 : Subsystem  DialogController=POWERSYS.PowerSysDialog  mask(Single-Phase Dynamic Load){NominalVoltage=|, ActiveReactivePowers=[330455.6138 202114.2565], PositiveSequence=[1 0], ExternalControl=on, NpNq=[np nq], TimeConstants=[0  0  0  0], MinimumVoltage=Vmin, LoadFlowParameters=[4,0,0,0,0]}
      mask NominalVoltage=|
      | [7967.4337
      | 60]
      mask prompts: NominalVoltage "Nominal voltage and frequency  [Vn(Vrms) fn(Hz)]:"; ActiveReactivePowers "Active and reactive power at initial voltage [Po(W) Qo(var)]:"; PositiveSequence "Initial voltage Vo [Mag(pu) Phase (deg.)]:"; ExternalControl "External control of PQ"; NpNq "Parameters [ np  nq ]:"; TimeConstants "Time constants [Tp1 Tp2 Tq1 Tq2]  (s):"; MinimumVoltage "Minimum voltage Vmin (pu):"; LoadFlowParameters "Load Flow parameters"
      mask help:
      | Implements a single-phase dynamic load. Active  power P and reactive
      | power Q absorbed by the load vary as function of voltage V  according to the
      | following equations:
      |
      |   If V>Vmin, P and Q vary as follows:
      |        P = Po * (V/Vo)^np * (1+Tp1.s)/(1+Tp2.s)
      |        Q = Qo * (V/Vo)^nq * (1+Tq1.s)/(1+Tq2.s)
      |   if V<Vmin
      |      Same equations with np=nq=2 (constant impedance load)
      mask init: same as Feeder_1/SM_NG/Single-Phase Dynamic Load32
      mask Help: helpview(psbhelp)
      mask Callback ExternalControl: powericon('ThreePhaseDynamicLoadCback',gcb);
      mask Display:
      | plot(-45,-45,45,45,[0,9,18,24,29,30,29,24,18,9,0,-9,-18,-24,-29,-30,-29,-24,-18,-9,0]*.9,[30,29,24,18,9,0,-9,-18,-24,-29,-30,-29,-24,-18,-9,0,9,18,24,29,30]*.9)
      | plot([0,0,10,0,-10,0]*1.1,[15,-5,-5,-15,-5,-5]*1.1)
  A : PMIOPort  Port=1  Side=Right
  B : PMIOPort  Port=2  Side=Right
  C : PMIOPort  Port=3  Side=Right
  wires:
  P/1 -> Single-Phase Dynamic Load2/1(P), Single-Phase Dynamic Load1/1(P), Single-Phase Dynamic Load9/1(P)
  Q/1 -> Single-Phase Dynamic Load1/2(Q), Single-Phase Dynamic Load2/2(Q), Single-Phase Dynamic Load9/2(Q)
  connections:
  Single-Phase Dynamic Load9/LConn2 -- Single-Phase Dynamic Load1/LConn2 -- Ground27/LConn1 -- Single-Phase Dynamic Load2/LConn2
  A/RConn1 -- Single-Phase Dynamic Load9/LConn1
  Single-Phase Dynamic Load2/LConn1 -- C/RConn1
  Single-Phase Dynamic Load1/LConn1 -- B/RConn1

== system Feeder_1/SM_NG/Dynamic Load BCDC4 ==
  P : Inport
  Q : Inport  Port=2
  Ground27 : powerlib/Elements/Ground  LConnTagsString=a
  Single-Phase Dynamic Load1 : Subsystem  DialogController=POWERSYS.PowerSysDialog  mask(Single-Phase Dynamic Load){NominalVoltage=|, ActiveReactivePowers=[359272.8363 164258.4315], PositiveSequence=[1 0], ExternalControl=on, NpNq=[np nq], TimeConstants=[0  0  0  0], MinimumVoltage=Vmin, LoadFlowParameters=[4,0,0,0,0]}
      mask NominalVoltage=|
      | [7967.4337
      | 60]
      mask prompts: NominalVoltage "Nominal voltage and frequency  [Vn(Vrms) fn(Hz)]:"; ActiveReactivePowers "Active and reactive power at initial voltage [Po(W) Qo(var)]:"; PositiveSequence "Initial voltage Vo [Mag(pu) Phase (deg.)]:"; ExternalControl "External control of PQ"; NpNq "Parameters [ np  nq ]:"; TimeConstants "Time constants [Tp1 Tp2 Tq1 Tq2]  (s):"; MinimumVoltage "Minimum voltage Vmin (pu):"; LoadFlowParameters "Load Flow parameters"
      mask help:
      | Implements a single-phase dynamic load. Active  power P and reactive
      | power Q absorbed by the load vary as function of voltage V  according to the
      | following equations:
      |
      |   If V>Vmin, P and Q vary as follows:
      |        P = Po * (V/Vo)^np * (1+Tp1.s)/(1+Tp2.s)
      |        Q = Qo * (V/Vo)^nq * (1+Tq1.s)/(1+Tq2.s)
      |   if V<Vmin
      |      Same equations with np=nq=2 (constant impedance load)
      mask init: same as Feeder_1/SM_NG/Single-Phase Dynamic Load32
      mask Help: helpview(psbhelp)
      mask Callback ExternalControl: powericon('ThreePhaseDynamicLoadCback',gcb);
      mask Display:
      | plot(-45,-45,45,45,[0,9,18,24,29,30,29,24,18,9,0,-9,-18,-24,-29,-30,-29,-24,-18,-9,0]*.9,[30,29,24,18,9,0,-9,-18,-24,-29,-30,-29,-24,-18,-9,0,9,18,24,29,30]*.9)
      | plot([0,0,10,0,-10,0]*1.1,[15,-5,-5,-15,-5,-5]*1.1)
  Single-Phase Dynamic Load2 : Subsystem  DialogController=POWERSYS.PowerSysDialog  mask(Single-Phase Dynamic Load){NominalVoltage=|, ActiveReactivePowers=[167826.2591 104736.8385], PositiveSequence=[1 0], ExternalControl=on, NpNq=[np nq], TimeConstants=[0  0  0  0], MinimumVoltage=Vmin, LoadFlowParameters=[4,0,0,0,0]}
      mask NominalVoltage=|
      | [7967.4337
      | 60]
      mask prompts: NominalVoltage "Nominal voltage and frequency  [Vn(Vrms) fn(Hz)]:"; ActiveReactivePowers "Active and reactive power at initial voltage [Po(W) Qo(var)]:"; PositiveSequence "Initial voltage Vo [Mag(pu) Phase (deg.)]:"; ExternalControl "External control of PQ"; NpNq "Parameters [ np  nq ]:"; TimeConstants "Time constants [Tp1 Tp2 Tq1 Tq2]  (s):"; MinimumVoltage "Minimum voltage Vmin (pu):"; LoadFlowParameters "Load Flow parameters"
      mask help:
      | Implements a single-phase dynamic load. Active  power P and reactive
      | power Q absorbed by the load vary as function of voltage V  according to the
      | following equations:
      |
      |   If V>Vmin, P and Q vary as follows:
      |        P = Po * (V/Vo)^np * (1+Tp1.s)/(1+Tp2.s)
      |        Q = Qo * (V/Vo)^nq * (1+Tq1.s)/(1+Tq2.s)
      |   if V<Vmin
      |      Same equations with np=nq=2 (constant impedance load)
      mask init: same as Feeder_1/SM_NG/Single-Phase Dynamic Load32
      mask Help: helpview(psbhelp)
      mask Callback ExternalControl: powericon('ThreePhaseDynamicLoadCback',gcb);
      mask Display:
      | plot(-45,-45,45,45,[0,9,18,24,29,30,29,24,18,9,0,-9,-18,-24,-29,-30,-29,-24,-18,-9,0]*.9,[30,29,24,18,9,0,-9,-18,-24,-29,-30,-29,-24,-18,-9,0,9,18,24,29,30]*.9)
      | plot([0,0,10,0,-10,0]*1.1,[15,-5,-5,-15,-5,-5]*1.1)
  Single-Phase Dynamic Load9 : Subsystem  DialogController=POWERSYS.PowerSysDialog  mask(Single-Phase Dynamic Load){NominalVoltage=|, ActiveReactivePowers=[330455.6138 202114.2565], PositiveSequence=[1 0], ExternalControl=on, NpNq=[np nq], TimeConstants=[0  0  0  0], MinimumVoltage=Vmin, LoadFlowParameters=[4,0,0,0,0]}
      mask NominalVoltage=|
      | [7967.4337
      | 60]
      mask prompts: NominalVoltage "Nominal voltage and frequency  [Vn(Vrms) fn(Hz)]:"; ActiveReactivePowers "Active and reactive power at initial voltage [Po(W) Qo(var)]:"; PositiveSequence "Initial voltage Vo [Mag(pu) Phase (deg.)]:"; ExternalControl "External control of PQ"; NpNq "Parameters [ np  nq ]:"; TimeConstants "Time constants [Tp1 Tp2 Tq1 Tq2]  (s):"; MinimumVoltage "Minimum voltage Vmin (pu):"; LoadFlowParameters "Load Flow parameters"
      mask help:
      | Implements a single-phase dynamic load. Active  power P and reactive
      | power Q absorbed by the load vary as function of voltage V  according to the
      | following equations:
      |
      |   If V>Vmin, P and Q vary as follows:
      |        P = Po * (V/Vo)^np * (1+Tp1.s)/(1+Tp2.s)
      |        Q = Qo * (V/Vo)^nq * (1+Tq1.s)/(1+Tq2.s)
      |   if V<Vmin
      |      Same equations with np=nq=2 (constant impedance load)
      mask init: same as Feeder_1/SM_NG/Single-Phase Dynamic Load32
      mask Help: helpview(psbhelp)
      mask Callback ExternalControl: powericon('ThreePhaseDynamicLoadCback',gcb);
      mask Display:
      | plot(-45,-45,45,45,[0,9,18,24,29,30,29,24,18,9,0,-9,-18,-24,-29,-30,-29,-24,-18,-9,0]*.9,[30,29,24,18,9,0,-9,-18,-24,-29,-30,-29,-24,-18,-9,0,9,18,24,29,30]*.9)
      | plot([0,0,10,0,-10,0]*1.1,[15,-5,-5,-15,-5,-5]*1.1)
  A : PMIOPort  Port=1  Side=Right
  B : PMIOPort  Port=2  Side=Right
  C : PMIOPort  Port=3  Side=Right
  wires:
  P/1 -> Single-Phase Dynamic Load2/1(P), Single-Phase Dynamic Load1/1(P), Single-Phase Dynamic Load9/1(P)
  Q/1 -> Single-Phase Dynamic Load1/2(Q), Single-Phase Dynamic Load2/2(Q), Single-Phase Dynamic Load9/2(Q)
  connections:
  Single-Phase Dynamic Load9/LConn2 -- Single-Phase Dynamic Load1/LConn2 -- Ground27/LConn1 -- Single-Phase Dynamic Load2/LConn2
  A/RConn1 -- Single-Phase Dynamic Load9/LConn1
  Single-Phase Dynamic Load2/LConn1 -- C/RConn1
  Single-Phase Dynamic Load1/LConn1 -- B/RConn1

== system Feeder_1/SM_NG/IED10 ==
  Current Measurement : powerlib/Measurements/Current Measurement  PhasorSimulation=off  OutputType=Complex  PSBequivalent=0
  Ground1 : powerlib/Elements/Ground  LConnTagsString=a
  Voltage Measurement : powerlib/Measurements/Voltage Measurement  PhasorSimulation=off  OutputType=Complex  PSBequivalent=0
  A : PMIOPort  Port=1  Side=Right
  a : PMIOPort  Port=2  Side=Left
  tag scope: I_IED10=global, V_IED10=global
  wires:
  Current Measurement/1 -> [I_IED10]
  Voltage Measurement/1 -> [V_IED10]
  connections:
  Ground1/LConn1 -- Voltage Measurement/LConn2
  Current Measurement/LConn1 -- a/RConn1
  Voltage Measurement/LConn1 -- A/RConn1 -- Current Measurement/RConn1

== system Feeder_1/SM_NG/IED14A ==
  Current Measurement : powerlib/Measurements/Current Measurement  PhasorSimulation=off  OutputType=Complex  PSBequivalent=0
  Ground1 : powerlib/Elements/Ground  LConnTagsString=a
  Voltage Measurement : powerlib/Measurements/Voltage Measurement  PhasorSimulation=off  OutputType=Complex  PSBequivalent=0
  A : PMIOPort  Port=1  Side=Right
  a : PMIOPort  Port=2  Side=Left
  tag scope: I_IED14A=global, V_IED14A=global
  wires:
  Current Measurement/1 -> [I_IED14A]
  Voltage Measurement/1 -> [V_IED14A]
  connections:
  Ground1/LConn1 -- Voltage Measurement/LConn2
  Current Measurement/LConn1 -- a/RConn1
  Voltage Measurement/LConn1 -- A/RConn1 -- Current Measurement/RConn1

== system Feeder_1/SM_NG/IED7A ==
  Current Measurement : powerlib/Measurements/Current Measurement  PhasorSimulation=off  OutputType=Complex  PSBequivalent=0
  Ground1 : powerlib/Elements/Ground  LConnTagsString=a
  Voltage Measurement : powerlib/Measurements/Voltage Measurement  PhasorSimulation=off  OutputType=Complex  PSBequivalent=0
  A : PMIOPort  Port=1  Side=Right
  a : PMIOPort  Port=2  Side=Left
  tag scope: I_IED7A=global, V_IED7A=global
  wires:
  Current Measurement/1 -> [I_IED7A]
  Voltage Measurement/1 -> [V_IED7A]
  connections:
  Ground1/LConn1 -- Voltage Measurement/LConn2
  Current Measurement/LConn1 -- a/RConn1
  Voltage Measurement/LConn1 -- A/RConn1 -- Current Measurement/RConn1

== system Feeder_1/SM_NG/PV11 ==
  PQ : Inport
  -Q : Gain  Gain=-1  SaturateOnIntegerOverflow=on  OutDataTypeStr=Inherit: Same as input  ParamDataTypeStr=Inherit: Same as input
  Dynamic Load : powerlib/Elements/Three-Phase Dynamic Load  NominalVoltage=[13800.00 60 ]  ActiveReactivePowers=|  PositiveSequence=[0.994 -11.8]  ExternalControl=on  NpNq=[np nq]  TimeConstants="[0  0  0  0]"  MinimumVoltage=Vmin  Tfilter=1e-4  LoadFlowParameters=[4,0,0,0,0]
      | [-684000.00
      | 0]
  a : PMIOPort  Port=1  Side=Right
  b : PMIOPort  Port=2  Side=Right
  c : PMIOPort  Port=3  Side=Right
  wires:
  PQ/1 -> -Q/1
  -Q/1 -> Dynamic Load/1
  connections:
  a/RConn1 -- Dynamic Load/LConn1
  c/RConn1 -- Dynamic Load/LConn3
  b/RConn1 -- Dynamic Load/LConn2

== system Feeder_1/SM_NG/Single-Phase Dynamic Load30 ==
  PQ : Inport
  Controlled Current Source : powerlib/Electrical Sources/Controlled Current Source  Initialize=on  Source_Type=AC  Amplitude=0  Phase=0  Frequency=0  Measurements=None
  Ground50 : powerlib/Elements/Ground  LConnTagsString=a
  Voltage Measurement1 : powerlib/Measurements/Voltage Measurement  PhasorSimulation=off  OutputType=Complex  PSBequivalent=0
  model : Subsystem
  a : PMIOPort  Tag=PMCPort  Port=1  Side=Right
  wires:
  PQ/1 -> model/2(PQ)
  Voltage Measurement1/1 -> model/1(v)
  model/1(i) -> Controlled Current Source/1
  connections:
  Controlled Current Source/RConn1 -- Voltage Measurement1/LConn1 -- a/RConn1
  Controlled Current Source/LConn1 -- Ground50/LConn1 -- Voltage Measurement1/LConn2

== system Feeder_1/SM_NG/Single-Phase Dynamic Load32 ==
  PQ : Inport
  Controlled Current Source : powerlib/Electrical Sources/Controlled Current Source  Initialize=on  Source_Type=AC  Amplitude=0  Phase=0  Frequency=0  Measurements=None
  Ground52 : powerlib/Elements/Ground  LConnTagsString=a
  Voltage Measurement1 : powerlib/Measurements/Voltage Measurement  PhasorSimulation=off  OutputType=Complex  PSBequivalent=0
  model : Subsystem
  a : PMIOPort  Tag=PMCPort  Port=1  Side=Right
  wires:
  PQ/1 -> model/2(PQ)
  Voltage Measurement1/1 -> model/1(v)
  model/1(i) -> Controlled Current Source/1
  connections:
  Voltage Measurement1/LConn1 -- a/RConn1 -- Controlled Current Source/RConn1
  Voltage Measurement1/LConn2 -- Controlled Current Source/LConn1 -- Ground52/LConn1

== system Feeder_1/SM_NG/Single-Phase Dynamic Load33 ==
  PQ : Inport
  Controlled Current Source : powerlib/Electrical Sources/Controlled Current Source  Initialize=on  Source_Type=AC  Amplitude=0  Phase=0  Frequency=0  Measurements=None
  Ground52 : powerlib/Elements/Ground  LConnTagsString=a
  Voltage Measurement1 : powerlib/Measurements/Voltage Measurement  PhasorSimulation=off  OutputType=Complex  PSBequivalent=0
  model : Subsystem
  a : PMIOPort  Tag=PMCPort  Port=1  Side=Right
  wires:
  PQ/1 -> model/2(PQ)
  Voltage Measurement1/1 -> model/1(v)
  model/1(i) -> Controlled Current Source/1
  connections:
  Voltage Measurement1/LConn1 -- a/RConn1 -- Controlled Current Source/RConn1
  Voltage Measurement1/LConn2 -- Ground52/LConn1 -- Controlled Current Source/LConn1

== system Feeder_1/SM_NG/Single-Phase Dynamic Load34 ==
  PQ : Inport
  Controlled Current Source : powerlib/Electrical Sources/Controlled Current Source  Initialize=on  Source_Type=AC  Amplitude=0  Phase=0  Frequency=0  Measurements=None
  Ground52 : powerlib/Elements/Ground  LConnTagsString=a
  Voltage Measurement1 : powerlib/Measurements/Voltage Measurement  PhasorSimulation=off  OutputType=Complex  PSBequivalent=0
  model : Subsystem
  a : PMIOPort  Tag=PMCPort  Port=1  Side=Right
  wires:
  PQ/1 -> model/2(PQ)
  Voltage Measurement1/1 -> model/1(v)
  model/1(i) -> Controlled Current Source/1
  connections:
  Voltage Measurement1/LConn1 -- a/RConn1 -- Controlled Current Source/RConn1
  Voltage Measurement1/LConn2 -- Ground52/LConn1 -- Controlled Current Source/LConn1

== system Feeder_1/SM_NG/Single-Phase Dynamic Load35 ==
  PQ : Inport
  Controlled Current Source : powerlib/Electrical Sources/Controlled Current Source  Initialize=on  Source_Type=AC  Amplitude=0  Phase=0  Frequency=0  Measurements=None
  Ground52 : powerlib/Elements/Ground  LConnTagsString=a
  Voltage Measurement1 : powerlib/Measurements/Voltage Measurement  PhasorSimulation=off  OutputType=Complex  PSBequivalent=0
  model : Subsystem
  a : PMIOPort  Tag=PMCPort  Port=1  Side=Right
  wires:
  PQ/1 -> model/2(PQ)
  Voltage Measurement1/1 -> model/1(v)
  model/1(i) -> Controlled Current Source/1
  connections:
  Voltage Measurement1/LConn1 -- a/RConn1 -- Controlled Current Source/RConn1
  Voltage Measurement1/LConn2 -- Controlled Current Source/LConn1 -- Ground52/LConn1
